simulink model "DC_Microgrid_Sim"  (R2023b)
settings: Solver=VariableStepDiscrete  StartTime=0.0  StopTime=720  MaxStep=1e2  RelTol=1e-3
undefined symbols (not defined in the file or in its folder): Ion, Lithium, Ts_Control, Ts_Power
libraries: spsDiodeLib x2, spsFirstOrderFilterLib x2, spsSeriesRLCBranchLib x2, SignalEditorBlockLib x2, spsBatteryLib x1, spsBoostConverterLib x1, spsCurrentMeasurementLib x1, spsStairGeneratorLib x1, spsPWMGeneratorPulseAveragingLib x1, spsPVArrayLib x1, spsVoltageMeasurementLib x1, spsVariableResistorLib x1
settings Model: SimulationMode=accelerator  Creator=andrewboland  LastModifiedBy=andrewboland

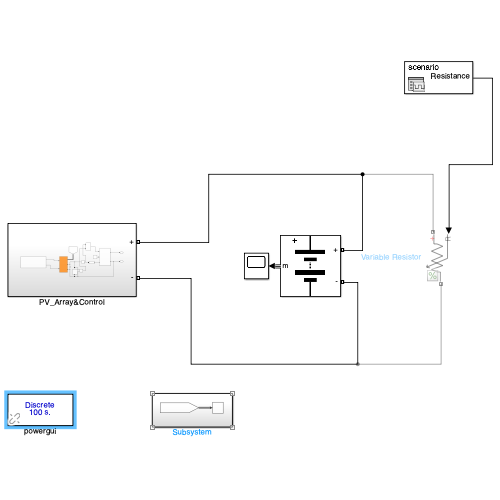
[thumbnail: Simulink's stored preview of the top-level diagram]
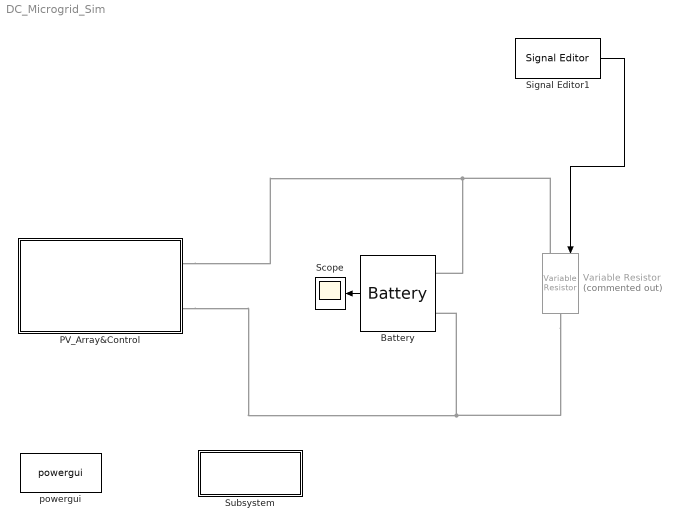
== system DC_Microgrid_Sim ==
  Battery : spsBatteryLib/Battery  BatType=Lithium-Ion  ShowTempParam=off  ThermalPreset=no  ShowAgeParam=off  NomV=200  NomQ=180  SOC=40  Batt_Tr=30  PresetModel=on  MaxQ=180  MinV=150  FullV=232.7974  Dis_rate=78.2609  R=0.011111  Normal_OP=162.7826  expZone="[216.0772      8.843478]"  current=[6.5 13 32.5]  Units=Time  Tci=20  NomT=20  T2=-30  MaxQ2=4.8  FullV2=7.1  Normal_OP2=5.655  expZone2="[6.58           1]"  Rca=0.6  ti=2000  Dp=0  Neq0=0  Tsim=1e6  Ta1=25  Qeol=5.4*0.9  Reol=0.013333*1.2  Char_age=[2.3478, 3]  Dis_age=[2.3478, 10]  N1=1500  N2=10500  N3=1000  N4=1400  Ta2=45  N5=950
  PV_Array&Control : Subsystem
  Scope : Scope
  Signal Editor1 : SignalEditorBlockLib/Signal Editor  FileName=/Users/andrewboland/Documents/MATLAB/Research/load_signal.mat  ActiveScenario=scenario  ActiveSignal=Resistance  IsBus=off  OutputBusObjectStr=Bus: BusObject  SampleTime=0  Interpolate=off  ZeroCross=off  OutputAfterFinalValue=Setting to zero  Unit=inherit  PreserveSignalName=on  ApplySigPropsToAllScenarios=on  ApplySigPropsToAllSignals=off
  Subsystem : Subsystem
  Variable Resistor : spsVariableResistorLib/Variable Resistor  Commented=on  Rabsmin=1e-3
      settings: LibrarySourceBlock=sps_lib/Passives/Variable Resistor
  powergui : sps_lib/powergui  Priority=1  SimulationMode=Discrete  SampleTime=1e2  frequency=60  Iterations=50  frequencyindice=0  Pbase=100e6  ErrMax=1e-4  UnitsV=kV  UnitsW=MW  buscounter=0  FunctionMessages=off  echomessages=off  EnableUseOfTLC=off  CurrentSourceSwitches=off  DisableSnubberDevices=off  DisableRonSwitches=off  DisableVfSwitches=off  DisplayEquations=off  AutomaticDiscreteSolvers=off  SolverType=Tustin/Backward Euler (TBE)  Interpol=off  ExternalGateDelay=off  methode=off  Ts=100  x0status=blocks  SPID=on  SwTol=0  HookPort=off  NonlinearTolerance=1e-4  nMaxIteration=100  ContinueOnMaxIteration=off  RestoreLinks=warning  ResistiveCurrentMeasurement=off  Frange=[0:2:500]  Ylog=off  Xlog=on  ShowGrid=off  save=off  variable=ZData  structure=0  ZoomFFT=off  StartTime=0.0  cycles=1  DisplayStyle=1  fundamental=60  FreqAxis=off  MaxFrequency=1000  frequencyindicesteady=1  RmsSteady=1  display=off
  wires:
  Battery/1 -> Scope/1
  Signal Editor1/1 -> Variable Resistor/1
  connections:
  Variable Resistor/LConn1 -- PV_Array&Control/RConn1 -- Battery/LConn1
  Variable Resistor/RConn1 -- PV_Array&Control/RConn2 -- Battery/LConn2

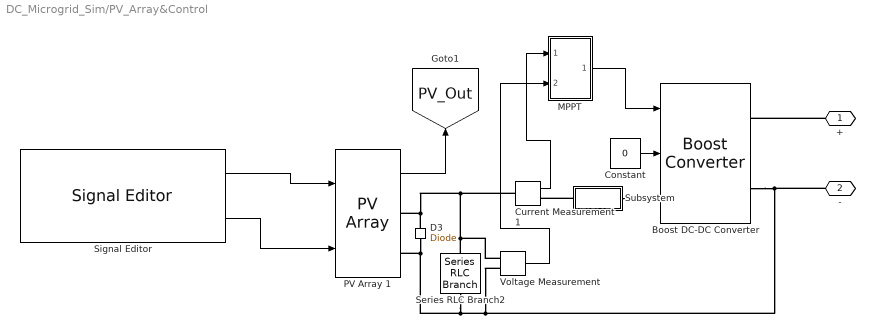
== system DC_Microgrid_Sim/PV_Array&Control ==
  Boost DC-DC Converter : spsBoostConverterLib/Boost Converter  ModelType=Switching function  Ron=1e-3  Rs=1e6  Cs=inf  Vforward=[0,0]  Ron_Diode=1e-3  Rs_Diode=1e6  Cs_Diode=inf  Vf_Diode=0  Rs_CurrentSource=inf  Ron_ACsource=1e-3
  Constant : Constant  Value=0
  Current Measurement1 : spsCurrentMeasurementLib/Current Measurement  PhasorSimulation=off  OutputType=Complex  PSBequivalent=0
  D3 : spsDiodeLib/Diode  Ron=1e-3  Lon=0  Vf=Vf_Diode  IC=0  UseSnubber=0  Rs=1e6  Cs=inf  Measurements=off
  MPPT : Subsystem
  PV Array 1 : spsPVArrayLib/PV Array  Npar=64  Nser=5  PlotType=array @ 1000 W/m2 & specified temperatures  S_vec="[ 1000  500  100 ]"  Temp_C_vec="[ 45 25  ]"  ModuleName=SunPower SPR-315E-WHT-D  PlotWhenSelected=off  Pm=315.072  Ncell=96  Voc=64.6  Isc=6.14  Vm=54.7  Im=5.76  beta_Voc_pc=-0.2727  alpha_Isc_pc=0.061743  beta_Voc=-0.17616  alpha_Isc=0.003791  IL=6.1461  I0=6.5067e-12  nI=0.95071  Rsh=430.0666  Rs=0.43041  RobustModel=off  RobustCellTemperature=40  BAL=on  Tc=1e-6  Tfilter=5e-5
  Series RLC Branch2 : spsSeriesRLCBranchLib/Series RLC Branch  LConnTagsString=__new0  RConnTagsString=__new0  BranchType=C  Resistance=10e-3  Inductance=10e-3  SetiL0=off  InitialCurrent=0  Capacitance=10e-6  Setx0=off  InitialVoltage=0  Measurements=None
  Signal Editor : SignalEditorBlockLib/Signal Editor  FileName=/Users/andrewboland/Documents/MATLAB/Research/pv_signals.mat  ActiveScenario=scenario  ActiveSignal=Irradiance  IsBus=off  OutputBusObjectStr=Bus: BusObject  SampleTime=0  Interpolate=off  ZeroCross=off  OutputAfterFinalValue=Setting to zero  Unit=inherit  PreserveSignalName=on  ApplySigPropsToAllScenarios=on  ApplySigPropsToAllSignals=off
  Subsystem : Subsystem
  Voltage Measurement : spsVoltageMeasurementLib/Voltage Measurement  PhasorSimulation=off  OutputType=Complex  PSBequivalent=0
  + : PMIOPort  Side=Right
  - : PMIOPort  Port=2  Side=Right
  tag scope: PV_Out=global
  wires:
  Signal Editor/1 -> PV Array 1/1
  PV Array 1/1 -> [PV_Out]
  Constant/1 -> Boost DC-DC Converter/2
  Current Measurement1/1 -> MPPT/1(In1)
  Voltage Measurement/1 -> MPPT/2(In2)
  MPPT/1(Out1) -> Boost DC-DC Converter/1
  Signal Editor/2 -> PV Array 1/2
  connections:
  Series RLC Branch2/LConn1 -- Voltage Measurement/LConn1 -- Current Measurement1/LConn1 -- D3/RConn1 -- PV Array 1/RConn1
  Boost DC-DC Converter/RConn2 -- -/RConn1 -- Voltage Measurement/LConn2 -- Series RLC Branch2/RConn1 -- D3/LConn1 -- PV Array 1/RConn2
  Subsystem/RConn1 -- Boost DC-DC Converter/LConn1
  Subsystem/LConn1 -- Current Measurement1/RConn1
  +/RConn1 -- Boost DC-DC Converter/RConn1

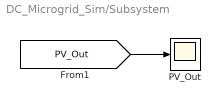
== system DC_Microgrid_Sim/Subsystem ==
  PV_Out : Scope
  wires:
  [PV_Out] -> PV_Out/1

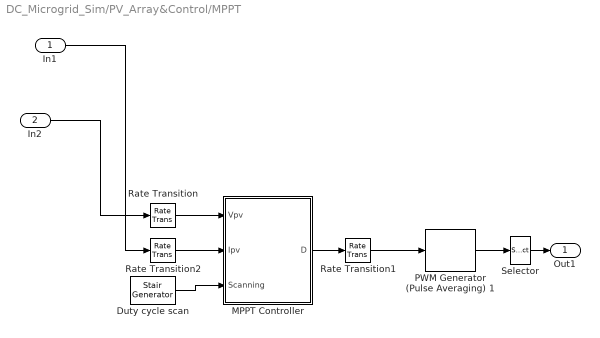
== system DC_Microgrid_Sim/PV_Array&Control/MPPT ==
  In1 : Inport
  In2 : Inport  Port=2
  Duty cycle scan : spsStairGeneratorLib/Stair Generator  t=[0,0.40, 0.41]  e=[0, 1, 0]  Ts=Ts_Control
  MPPT Controller : Subsystem  mask(MPPT Controller - Perturb and Observe algorithm (PandO)){Dinit=0.39, Dlimits=[0.85, 0.30], deltaD=50e-6, Fc=1000, ScanDuration=0.25, Ts=Ts_Control}
      mask prompts: Dinit "Duty cycle (D) initial value"; Dlimits "D limits [Upper, Lower]"; deltaD "Increment value for PandO algorithm"; Fc "Measurement filter cutoff frequency (Hz)"; ScanDuration "Scanning mode duration (s)"; Ts "Sample time (s)"
      mask init:
      | Dmax=Dlimits(1);
      | Dmin=Dlimits(2);
      | SampleTime=Ts;
      | DeltaD_Scan=(Dmax-Dmin)*Ts/ScanDuration;
  PWM Generator (Pulse Averaging) 1 : spsPWMGeneratorPulseAveragingLib/PWM Generator (Pulse Averaging)  GeneratorType=Two-quadrant  Fc=20e3  InitialPhase=90  Ts=Ts_Power
  Rate Transition : RateTransition  OutPortSampleTime=Ts_Control
  Rate Transition1 : RateTransition  OutPortSampleTime=Ts_Power
  Rate Transition2 : RateTransition  OutPortSampleTime=Ts_Control
  Selector : Selector  InputPortWidth=2  IndexOptions=Index vector (dialog)  Indices=1  OutputSizes=1
  Out1 : Outport
  wires:
  Selector/1 -> Out1/1
  Rate Transition2/1 -> MPPT Controller/2(Ipv)
  In1/1 -> Rate Transition2/1
  In2/1 -> Rate Transition/1
  Rate Transition1/1 -> PWM Generator (Pulse Averaging) 1/1
  MPPT Controller/1(D) -> Rate Transition1/1
  Duty cycle scan/1 -> MPPT Controller/3(Scanning)
  Rate Transition/1 -> MPPT Controller/1(Vpv)
  PWM Generator (Pulse Averaging) 1/1 -> Selector/1

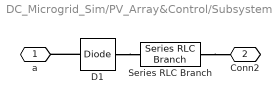
== system DC_Microgrid_Sim/PV_Array&Control/Subsystem ==
  D1 : spsDiodeLib/Diode  Ron=1e-3  Lon=0  Vf=Vf_Diode  IC=0  UseSnubber=0  Rs=1e6  Cs=inf  Measurements=off
  Series RLC Branch : spsSeriesRLCBranchLib/Series RLC Branch  LConnTagsString=__new0  RConnTagsString=__new0  BranchType=RL  Resistance=20e-3  Inductance=20e-3  SetiL0=off  InitialCurrent=0  Capacitance=1e-6  Setx0=off  InitialVoltage=0  Measurements=None
  a : PMIOPort  Side=Left
  Conn2 : PMIOPort  Port=2  Side=Right
  connections:
  D1/LConn1 -- a/RConn1
  Series RLC Branch/RConn1 -- Conn2/RConn1
  D1/RConn1 -- Series RLC Branch/LConn1

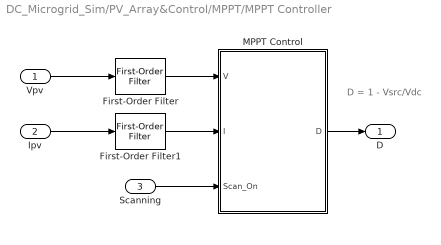
== system DC_Microgrid_Sim/PV_Array&Control/MPPT/MPPT Controller ==
  note: D = 1 - Vsrc/Vdc
  Vpv : Inport
  Ipv : Inport  Port=2
  Scanning : Inport  Port=3  PortDimensions=1
  First-Order Filter : spsFirstOrderFilterLib/First-Order Filter  FilterType=Lowpass  Tc=1/Fc  Ts=Ts  Initialize=off  Vac_Init=[0, 0, 60]  Vdc_Init=0  PlotResponse=off  FreqRange="[0,  200,  1]"
  First-Order Filter1 : spsFirstOrderFilterLib/First-Order Filter  FilterType=Lowpass  Tc=1/Fc  Ts=Ts  Initialize=off  Vac_Init=[0, 0, 60]  Vdc_Init=0  PlotResponse=off  FreqRange="[0,  200,  1]"
  MPPT Control : MATLAB Function  TreatAsAtomicUnit=on
  D : Outport  OutDataTypeStr=double  PortDimensions=1  VectorParamsAs1DForOutWhenUnconnected=off
  wires:
  First-Order Filter1/1 -> MPPT Control/2(I)
  First-Order Filter/1 -> MPPT Control/1(V)
  Ipv/1 -> First-Order Filter1/1
  Vpv/1 -> First-Order Filter/1
  MPPT Control/1(D) -> D/1
  Scanning/1 -> MPPT Control/3(Scan_On)

== matlab function DC_Microgrid_Sim/PV_Array&Control/MPPT/MPPT Controller/MPPT Control ==
  settings: updateMethod=DISCRETE  sampleTime=Ts
  data: V input =V; I input; D output; Dmax parameter; Dmin parameter; deltaD parameter; Dinit parameter; Scan_On input; DeltaD_Scan parameter
function D   = PandO(V, I, Dmax, Dmin, deltaD, Dinit, Scan_On, DeltaD_Scan)

% MPPT controller based on the Perturb & Observe algorithm.

% D output = Duty cycle of the boost converter (value between 0 and 1)
% V input = PV array terminal voltage (V)
% I input = PV array current (A)
% D = 1 - Vinput/Voutput (increasing D decrease Vin)

persistent Vold Pold Dold Scan_On_Old Pmax D_Pmax V_Pmax;
%
if isempty(Vold)
    Vold=0;
    Pold=0;
    Scan_On_Old=0;
    Dold=Dinit;
    Pmax=0;
    D_Pmax=0;
    V_Pmax=0;
end
P= V*I;
if Scan_On==1 || Scan_On_Old==1
    if Scan_On_Old==0
        Scan_On_Old=1;
        D=Dmin;
    else
        D=Dold+DeltaD_Scan;
    end
    Dold=D;
    if P>Pmax
        Pmax=P;
        D_Pmax=D;
    end
    if D >= Dmax
        Scan_On_Old=0;
        Pold=Pmax;
        Dold=D_Pmax;
        Vold=V_Pmax;
    end
else
    dV= V - Vold;
    dP= P - Pold;
    %
    if dP ~= 0
        if dP < 0
            if dV < 0
                D = Dold - deltaD;
            else
                D = Dold + deltaD;
            end
        else
            if dV < 0
                D = Dold + deltaD;
            else
                D = Dold - deltaD;
            end
        end
    else
        D=Dold;
    end
    %
    if D >= Dmax || D<= Dmin
        D=Dold;
    end
    %
    Dold=D;
    Vold=V;
    Pold=P;
end
